simulink model "Model"  (R2018a)
settings: Solver=ode4  StartTime=0.0  StopTime=100  FixedStep=0.001  RelTol=1e-3
values from neighbouring files (symbols this model uses):
  Delay = 0.1530    (= 0.153)    [CPA.m]
  den = [9.9926 1]    [CPA.m]
  Noise = 0.0    (= 0)    [CPA.m]
  num = -4.5753    [CPA.m]
settings Model: Creator=bizagi.las  LastModifiedBy=Rafael
settings CodeAppCC: StateflowObjectComments=on

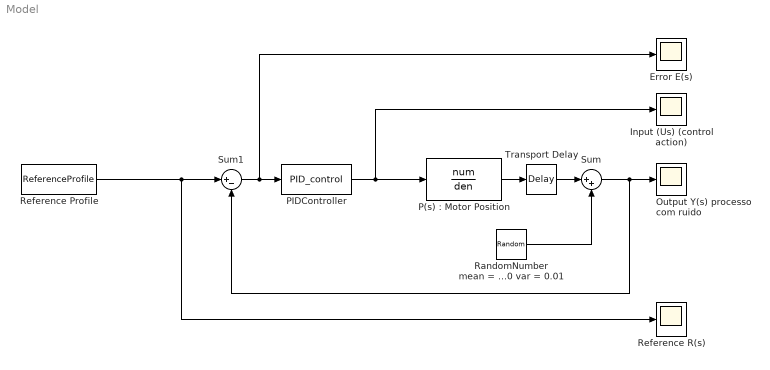
== system Model ==
  Error E(s) : Scope
  Input (Us) (control action) : Scope
  Output Y(s) processo com ruido : Scope
  "P(s) : Motor Position" : TransferFcn  Numerator=num  Denominator=den
  PIDController : MATLABFcn  MATLABFcn=PID_control  SampleTime=1/1000
  RandomNumber mean = 0 var = 0.01 : RandomNumber  Variance=Noise  SampleTime=0.001
  Reference Profile : FromWorkspace  VariableName=ReferenceProfile  SampleTime=0
  Reference R(s) : Scope
  Sum : Sum  Inputs=|++
  Sum1 : Sum  Inputs=|+-
  Transport Delay : TransportDelay  DelayTime=Delay
  wires:
  Sum/1 -> Sum1/2, Output Y(s) processo com ruido/1
  Sum1/1 -> Error E(s)/1, PIDController/1
  Reference Profile/1 -> Reference R(s)/1, Sum1/1
  PIDController/1 -> "P(s) : Motor Position"/1, Input (Us) (control action)/1
  RandomNumber mean = 0 var = 0.01/1 -> Sum/2
  "P(s) : Motor Position"/1 -> Transport Delay/1
  Transport Delay/1 -> Sum/1
